simulink model "trajgen_vel"  (R2021a)
settings: Solver=FixedStepDiscrete  StartTime=0.0  StopTime=10  RelTol=1e-3  EnableMultiTasking=on
settings Model: Creator=ihout_000  LastModifiedBy=ihout
settings SolverCC: AlgebraicLoopSolver=TrustRegion
settings DataIOCC: LimitDataPoints=on  SaveFormat=Array
settings OptimizationCC: ExpressionDepthLimit=2147483647  LifeSpan=inf  SimCompilerOptimization=on
settings DebuggingCC: SolverPrmCheckMsg=warning  StateNameClashWarn=warning  SFUnexpectedBacktrackingDiag=warning  SFNoUnconditionalDefaultTransitionDiag=warning  SFExecutionAtInitializationDiag=none  ArithmeticOperatorsInVariantConditions=warning
settings ModelReferenceCC: UpdateModelReferenceTargets=Force  PropagateSignalLabelsOutOfModel=off
settings SFSimCC: SimUserIncludeDirs=ReflexxesTypeII\include\  SimUseLocalCustomCode=off  CustomCodeUndefinedFunction=UseInterfaceOnly  SimTargetLang=C++
settings SFSimCC: SimUserSources=|
  | ReflexxesTypeII\src\TypeIIRML\ReflexxesAPI.cpp
  | ReflexxesTypeII\src\TypeIIRML\TypeIIRMLCalculatePositionalExtrems.cpp
  | ReflexxesTypeII\src\TypeIIRML\TypeIIRMLDecisions.cpp
  | ReflexxesTypeII\src\TypeIIRML\TypeIIRMLDecisionTree1A.cpp
  | ReflexxesTypeII\src\TypeIIRML\TypeIIRMLDecisionTree1B.cpp
  | ReflexxesTypeII\src\TypeIIRML\TypeIIRMLDecisionTree1C.cpp
  | ReflexxesTypeII\src\TypeIIRML\TypeIIRMLDecisionTree2.cpp
  | ReflexxesTypeII\src\TypeIIRML\TypeIIRMLFallBackStrategy.cpp
  | ReflexxesTypeII\src\TypeIIRML\TypeIIRMLIsPhaseSynchronizationPossible.cpp
  | ReflexxesTypeII\src\TypeIIRML\TypeIIRMLPolynomial.cpp
  | ReflexxesTypeII\src\TypeIIRML\TypeIIRMLPosition.cpp
  | ReflexxesTypeII\src\TypeIIRML\TypeIIRMLQuicksort.cpp
  | ReflexxesTypeII\src\TypeIIRML\TypeIIRMLSetupModifiedSelectionVector.cpp
  | ReflexxesTypeII\src\TypeIIRML\TypeIIRMLStep1.cpp
  | ReflexxesTypeII\src\TypeIIRML\TypeIIRMLStep1IntermediateProfiles.cpp
  | ReflexxesTypeII\src\TypeIIRML\TypeIIRMLStep1Profiles.cpp
  | ReflexxesTypeII\src\TypeIIRML\TypeIIRMLStep2.cpp
  | ReflexxesTypeII\src\TypeIIRML\TypeIIRMLStep2IntermediateProfiles.cpp
  | ReflexxesTypeII\src\TypeIIRML\TypeIIRMLStep2PhaseSynchronization.cpp
  | ReflexxesTypeII\src\TypeIIRML\TypeIIRMLStep2Profiles.cpp
  | ReflexxesTypeII\src\TypeIIRML\TypeIIRMLStep2WithoutSynchronization.cpp
  | ReflexxesTypeII\src\TypeIIRML\TypeIIRMLStep3.cpp
  | ReflexxesTypeII\src\TypeIIRML\TypeIIRMLVelocity.cpp
  | ReflexxesTypeII\src\TypeIIRML\TypeIIRMLVelocityCalculatePositionalExtrems.cpp
  | ReflexxesTypeII\src\TypeIIRML\TypeIIRMLVelocityFallBackStrategy.cpp
  | ReflexxesTypeII\src\TypeIIRML\TypeIIRMLVelocityIsPhaseSynchronizationPossible.cpp
  | ReflexxesTypeII\src\TypeIIRML\TypeIIRMLVelocityMethods.cpp
  | ReflexxesTypeII\src\TypeIIRML\TypeIIRMLVelocitySetupPhaseSyncSelectionVector.cpp
settings RTWCC: RTWUseLocalCustomCode=off  CustomInclude=ReflexxesTypeII\include\  Toolchain=Microsoft Visual C++ 2019 v16.0 | nmake (64-bit Windows)  BuildConfiguration=Faster Runs  TargetLang=C++  DLArmComputeVersion=20.02.1
settings RTWCC: CustomSource=|
  | ReflexxesTypeII\src\TypeIIRML\ReflexxesAPI.cpp
  | ReflexxesTypeII\src\TypeIIRML\TypeIIRMLCalculatePositionalExtrems.cpp
  | ReflexxesTypeII\src\TypeIIRML\TypeIIRMLDecisions.cpp
  | ReflexxesTypeII\src\TypeIIRML\TypeIIRMLDecisionTree1A.cpp
  | ReflexxesTypeII\src\TypeIIRML\TypeIIRMLDecisionTree1B.cpp
  | ReflexxesTypeII\src\TypeIIRML\TypeIIRMLDecisionTree1C.cpp
  | ReflexxesTypeII\src\TypeIIRML\TypeIIRMLDecisionTree2.cpp
  | ReflexxesTypeII\src\TypeIIRML\TypeIIRMLFallBackStrategy.cpp
  | ReflexxesTypeII\src\TypeIIRML\TypeIIRMLIsPhaseSynchronizationPossible.cpp
  | ReflexxesTypeII\src\TypeIIRML\TypeIIRMLPolynomial.cpp
  | ReflexxesTypeII\src\TypeIIRML\TypeIIRMLPosition.cpp
  | ReflexxesTypeII\src\TypeIIRML\TypeIIRMLQuicksort.cpp
  | ReflexxesTypeII\src\TypeIIRML\TypeIIRMLSetupModifiedSelectionVector.cpp
  | ReflexxesTypeII\src\TypeIIRML\TypeIIRMLStep1.cpp
  | ReflexxesTypeII\src\TypeIIRML\TypeIIRMLStep1IntermediateProfiles.cpp
  | ReflexxesTypeII\src\TypeIIRML\TypeIIRMLStep1Profiles.cpp
  | ReflexxesTypeII\src\TypeIIRML\TypeIIRMLStep2.cpp
  | ReflexxesTypeII\src\TypeIIRML\TypeIIRMLStep2IntermediateProfiles.cpp
  | ReflexxesTypeII\src\TypeIIRML\TypeIIRMLStep2PhaseSynchronization.cpp
  | ReflexxesTypeII\src\TypeIIRML\TypeIIRMLStep2Profiles.cpp
  | ReflexxesTypeII\src\TypeIIRML\TypeIIRMLStep2WithoutSynchronization.cpp
  | ReflexxesTypeII\src\TypeIIRML\TypeIIRMLStep3.cpp
  | ReflexxesTypeII\src\TypeIIRML\TypeIIRMLVelocity.cpp
  | ReflexxesTypeII\src\TypeIIRML\TypeIIRMLVelocityCalculatePositionalExtrems.cpp
  | ReflexxesTypeII\src\TypeIIRML\TypeIIRMLVelocityFallBackStrategy.cpp
  | ReflexxesTypeII\src\TypeIIRML\TypeIIRMLVelocityIsPhaseSynchronizationPossible.cpp
  | ReflexxesTypeII\src\TypeIIRML\TypeIIRMLVelocityMethods.cpp
  | ReflexxesTypeII\src\TypeIIRML\TypeIIRMLVelocitySetupPhaseSyncSelectionVector.cpp
settings CodeAppCC: StateflowObjectComments=on
settings GRTTargetCC: TargetLangStandard=C++03 (ISO)
settings ConfigComp: CovMetricSettings=dw  CovSaveCumulativeToWorkspaceVar=on  CovSaveSingleToWorkspaceVar=on  CovExternalEMLEnable=off  CovBoundaryAbsTol=1.0e-5

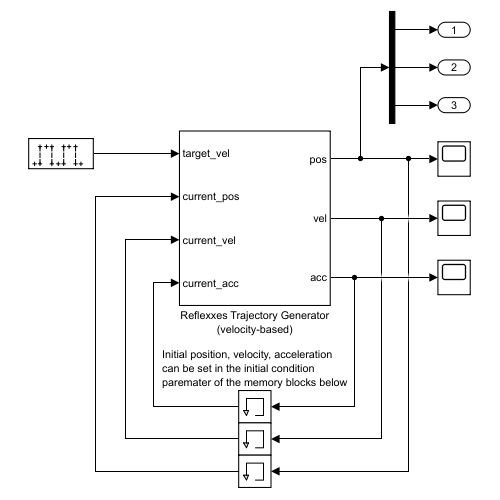
[thumbnail: Simulink's stored preview of the top-level diagram]
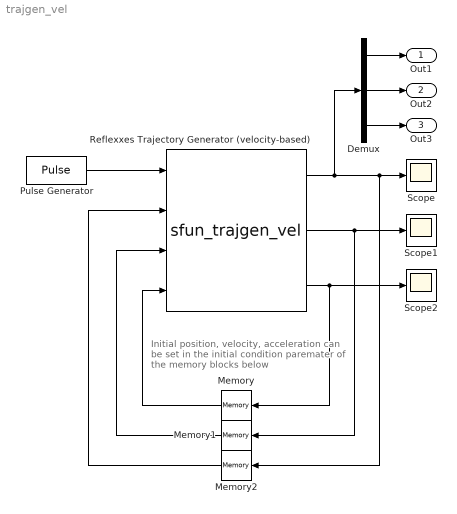
== system trajgen_vel ==
  note: Initial position, velocity, acceleration
      | can be set in the initial condition
      | paremater of the memory blocks below
  Demux : Demux  Outputs=3
  Memory : Memory  InitialCondition=[0 0 0]  InheritSampleTime=on
  Memory1 : Memory  InitialCondition=[0 0 0]  InheritSampleTime=on
  Memory2 : Memory  InitialCondition=[2 -1 1]  InheritSampleTime=on
  Pulse Generator : DiscretePulseGenerator  Amplitude=[150; 75; 100]  Period=500  PulseWidth=200  SampleTime=0.01
  Reflexxes Trajectory Generator (velocity-based) : S-Function  FunctionName=sfun_trajgen_vel  Parameters=ts,ndofs,amax,jmax,sync  SFunctionDeploymentMode=off  EnableBusSupport=off  mask{ts=1e-2, ndofs=3, amax=[500 500 1000], jmax=[500 1000 700], sync=NO_SYNCHRONIZATION}
      mask prompts: ts "Sample Time:"; ndofs "Number of DoF's:"; amax "Maximum Acceleration Vector:"; jmax "Maximum Jerk Vector:"; sync "Synchronization Behavior:"
      mask TypeOptions sync: NO_SYNCHRONIZATION | PHASE_SYNCHRONIZATION_IF_POSSIBLE | ONLY_TIME_SYNCHRONIZATION | ONLY_PHASE_SYNCHRONIZATION
      mask Display:
      | port_label('input', 1, 'target_vel')
      | port_label('input', 2, 'current_pos')
      | port_label('input', 3, 'current_vel')
      | port_label('input', 4, 'current_acc')
      | port_label('output', 1, 'pos')
      | port_label('output', 2, 'vel')
      | port_label('output', 3, 'acc')
  Scope : Scope
  Scope1 : Scope
  Scope2 : Scope
  Out1 : Outport  VectorParamsAs1DForOutWhenUnconnected=off
  Out2 : Outport  Port=2  VectorParamsAs1DForOutWhenUnconnected=off
  Out3 : Outport  Port=3  VectorParamsAs1DForOutWhenUnconnected=off
  wires:
  Pulse Generator/1 -> Reflexxes Trajectory Generator (velocity-based)/1
  Reflexxes Trajectory Generator (velocity-based)/1 -> Demux/1, Memory2/1, Scope/1
  Reflexxes Trajectory Generator (velocity-based)/2 -> Memory1/1, Scope1/1
  Reflexxes Trajectory Generator (velocity-based)/3 -> Scope2/1, Memory/1
  Demux/1 -> Out1/1
  Demux/2 -> Out2/1
  Demux/3 -> Out3/1
  Memory/1 -> Reflexxes Trajectory Generator (velocity-based)/4
  Memory1/1 -> Reflexxes Trajectory Generator (velocity-based)/3
  Memory2/1 -> Reflexxes Trajectory Generator (velocity-based)/2
